simulink subsystem "CO2_dissociation"  (R2020b)
settings: Solver=VariableStepAuto  StartTime=0.0  StopTime=10.0  RelTol=1e-3
settings Model: Creator=RH  LastModifiedBy=Marco

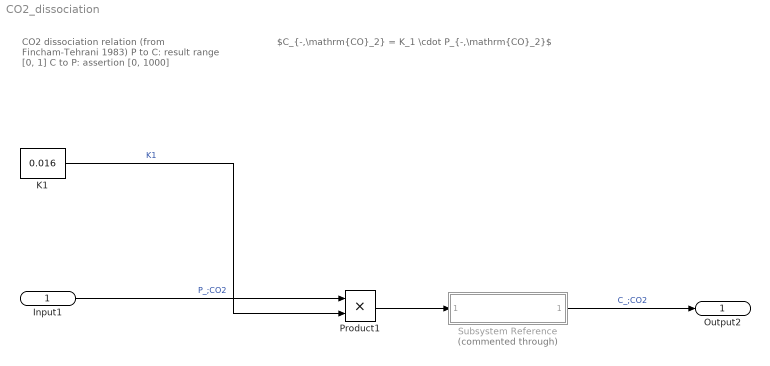
== system CO2_dissociation ==
  note: $C_{-,\mathrm{CO}_2} = K_1 \cdot P_{-,\mathrm{CO}_2}$
  note: CO2 dissociation relation
      | (from Fincham-Tehrani 1983)
      |
      | P to C: result range [0, 1]
      | C to P: assertion [0, 1000]
  Input1 : Inport  Unit=mmHg
  K1 : Constant  Value=0.016
  Product1 : Product
  Subsystem Reference : Subsystem  Commented=through  ReferencedSubsystem=saturation_range
  Output2 : Outport  Unit=1
  wires:
  Product1/1 -> Subsystem Reference/1
  Input1/1 -> Product1/1  "P_;CO2"
  Subsystem Reference/1 -> Output2/1  "C_;CO2"
  K1/1 -> Product1/2  "K1"
